simulink model "MOD1_CT"  (R2017a)
settings: Solver=FixedStepAuto  StartTime=0.0  StopTime=0.1  RelTol=1e-3  EnableMultiTasking=on
libraries: dspmlti4 x2, dsparch4 x1
settings Model: Creator=bhannigan  LastModifiedBy=bhannigan
settings OptimizationCC: LifeSpan=inf
settings DebuggingCC: SFUnexpectedBacktrackingDiag=warning  SFNoUnconditionalDefaultTransitionDiag=warning  SFExecutionAtInitializationDiag=none
settings GRTTargetCC: TargetLangStandard=C89/C90 (ANSI)  GeneratePreprocessorConditionals=Disable all
settings ConfigComp: CovMetricSettings=dw  CovHtmlReporting=on  CovSaveCumulativeToWorkspaceVar=on  CovSaveSingleToWorkspaceVar=on  CovExternalEMLEnable=off

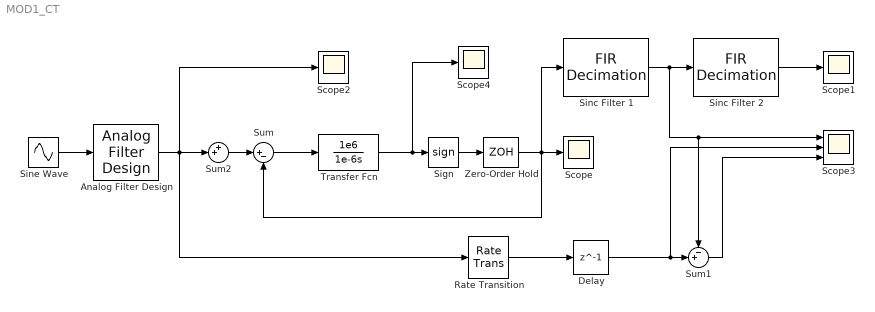
== system MOD1_CT ==
  Analog Filter Design : dsparch4/Analog Filter Design  method=Butterworth  filttype=Lowpass  N=5  Wlo=2*pi*2500  Whi=80  Rp=2  Rs=40
  Delay : Delay  DelayLength=1
  Rate Transition : RateTransition
  Scope{,1..2,4} (4 alike) : Scope
  Scope3 : Scope  NumInputPorts=3
  Sign : Signum
  Sinc Filter 1 : dspmlti4/FIR Decimation  FilterSource=Dialog parameters  h=1/64*ones(1, 64)  D=64  filtStruct=Direct form  FilterObject=FDECIM  framing=Enforce single-rate processing  inputOffset=0  outputBufInitCond=0  roundingMode=Floor  overflowMode=off  firstCoeffDataTypeStr=Inherit: Same word length as input  firstCoeffMin=[]  firstCoeffMax=[]  firstCoeffLastDataTypeStr=Inherit: Same word length as input  outputDataTypeStr=Inherit: Same as accumulator  outputMin=[]  outputMax=[]  outputLastDataTypeStr=Inherit: Same as accumulator
  Sinc Filter 2 : dspmlti4/FIR Decimation  FilterSource=Dialog parameters  h=1/64*ones(1, 64)  D=8  filtStruct=Direct form  FilterObject=FDECIM  framing=Enforce single-rate processing  inputOffset=0  outputBufInitCond=0  roundingMode=Floor  overflowMode=off  firstCoeffDataTypeStr=Inherit: Same word length as input  firstCoeffMin=[]  firstCoeffMax=[]  firstCoeffLastDataTypeStr=Inherit: Same word length as input  outputDataTypeStr=Inherit: Same as accumulator  outputMin=[]  outputMax=[]  outputLastDataTypeStr=Inherit: Same as accumulator
  Sine Wave : Sin  Frequency=2*pi*100  SampleTime=0
  Sum : Sum  Inputs=|+-
  Sum1 : Sum  Inputs=-+|
  Sum2 : Sum  Inputs=++|
  Transfer Fcn : TransferFcn  Numerator=1e6  Denominator=[1e-6 0]
  Zero-Order Hold : ZeroOrderHold  SampleTime=1/160000
  wires:
  Sine Wave/1 -> Analog Filter Design/1
  Sinc Filter 1/1 -> Scope3/1, Sum1/1, Sinc Filter 2/1
  Sinc Filter 2/1 -> Scope1/1
  Sign/1 -> Zero-Order Hold/1
  Analog Filter Design/1 -> Sum2/2, Scope2/1, Rate Transition/1
  Rate Transition/1 -> Delay/1
  Delay/1 -> Scope3/2, Sum1/2
  Sum1/1 -> Scope3/3
  Zero-Order Hold/1 -> Sum/2, Sinc Filter 1/1, Scope/1
  Sum2/1 -> Sum/1
  Sum/1 -> Transfer Fcn/1
  Transfer Fcn/1 -> Scope4/1, Sign/1
